simulink model "bai3c_pid"  (R2018a)
settings: Solver=VariableStepAuto  StartTime=0.0  StopTime=500  RelTol=1e-3
libraries: simulink x3
settings Model: Creator=MY PC  LastModifiedBy=Administrator
settings DataIOCC: ReturnWorkspaceOutputs=on
settings SFSimCC: SimUseLocalCustomCode=on
settings RTWCC: RTWUseLocalCustomCode=on

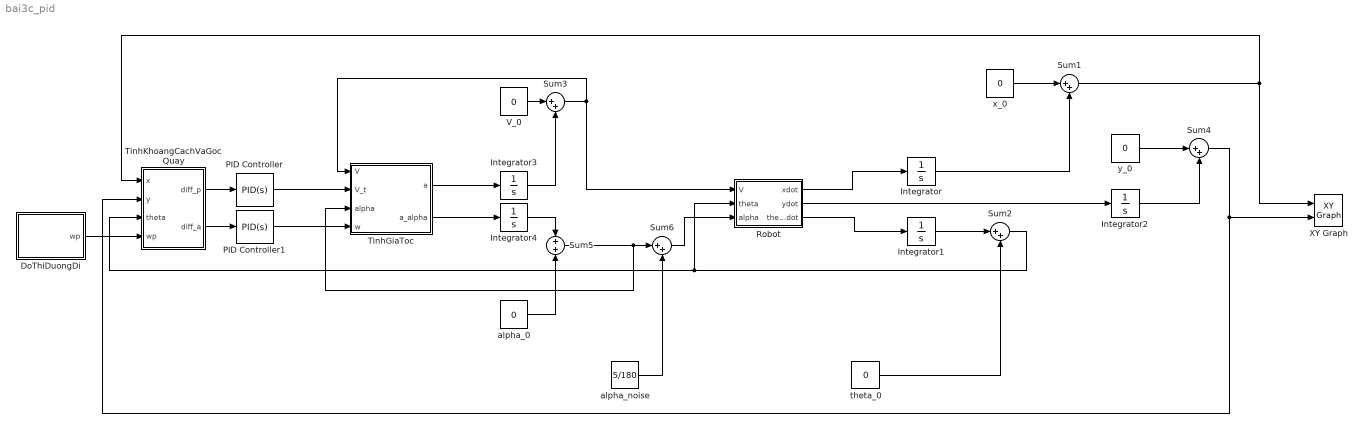
== system bai3c_pid ==
  DoThiDuongDi : MATLAB Function  TreatAsAtomicUnit=on
  Integrator{,1..4} (5 alike) : Integrator
  PID Controller : simulink/Continuous/PID Controller  Controller=PID  TimeDomain=Continuous-time  SampleTime=-1  IntegratorMethod=Forward Euler  FilterMethod=Forward Euler  Form=Parallel  UseFilter=on  ControllerParametersSource=internal  P=1/200  I=1/90000  D=0  N=1000000  InitialConditionSource=internal  InitialConditionForIntegrator=0  InitialConditionForFilter=0  ExternalReset=none  LimitOutput=off  UpperSaturationLimit=inf  LowerSaturationLimit=-inf  LinearizeAsGain=on  AntiWindupMode=none  Kb=1  TrackingMode=off  Kt=1  PParamMin=[]  PParamMax=[]  IParamMin=[]  IParamMax=[]  DParamMin=[]  DParamMax=[]  NParamMin=[]  NParamMax=[]  KbParamMin=[]  KbParamMax=[]  KtParamMin=[]  KtParamMax=[]  POutMin=[]  POutMax=[]  IOutMin=[]  IOutMax=[]  DOutMin=[]  DOutMax=[]  NOutMin=[]  NOutMax=[]  KbOutMin=[]  KbOutMax=[]  KtOutMin=[]  KtOutMax=[]  IntegratorOutMin=[]  IntegratorOutMax=[]  FilterOutMin=[]  FilterOutMax=[]  SumOutMin=[]  SumOutMax=[]  SumI1OutMin=[]  SumI1OutMax=[]  SumI2OutMin=[]  SumI2OutMax=[]  SumI3OutMin=[]  SumI3OutMax=[]  SumDOutMin=[]  SumDOutMax=[]  SaturationOutMin=[]  SaturationOutMax=[]  IntegratorContinuousStateAttributes=''  IntegratorStateMustResolveToSignalObject=off  IntegratorRTWStateStorageClass=Auto  FilterContinuousStateAttributes=''  FilterStateMustResolveToSignalObject=off  FilterRTWStateStorageClass=Auto  DifferentiatorICPrevScaledInput=0  DifferentiatorOutMin=[]  DifferentiatorOutMax=[]  FilterDiffOutCoefMin=[]  FilterDiffOutCoefMax=[]  SumDenOutMin=[]  SumDenOutMax=[]  SumNumOutMin=[]  SumNumOutMax=[]  ReciprocalOutMin=[]  ReciprocalOutMax=[]  DivideOutMin=[]  DivideOutMax=[]  TunerSelectOption=Transfer Function Based (PID Tuner App)
  PID Controller1 : simulink/Continuous/PID Controller  Controller=PID  TimeDomain=Continuous-time  SampleTime=-1  IntegratorMethod=Forward Euler  FilterMethod=Forward Euler  Form=Parallel  UseFilter=on  ControllerParametersSource=internal  P=1/10  I=0  D=0  N=10000  InitialConditionSource=internal  InitialConditionForIntegrator=0  InitialConditionForFilter=0  ExternalReset=none  LimitOutput=off  UpperSaturationLimit=inf  LowerSaturationLimit=-inf  LinearizeAsGain=on  AntiWindupMode=none  Kb=1  TrackingMode=off  Kt=1  PParamMin=[]  PParamMax=[]  IParamMin=[]  IParamMax=[]  DParamMin=[]  DParamMax=[]  NParamMin=[]  NParamMax=[]  KbParamMin=[]  KbParamMax=[]  KtParamMin=[]  KtParamMax=[]  POutMin=[]  POutMax=[]  IOutMin=[]  IOutMax=[]  DOutMin=[]  DOutMax=[]  NOutMin=[]  NOutMax=[]  KbOutMin=[]  KbOutMax=[]  KtOutMin=[]  KtOutMax=[]  IntegratorOutMin=[]  IntegratorOutMax=[]  FilterOutMin=[]  FilterOutMax=[]  SumOutMin=[]  SumOutMax=[]  SumI1OutMin=[]  SumI1OutMax=[]  SumI2OutMin=[]  SumI2OutMax=[]  SumI3OutMin=[]  SumI3OutMax=[]  SumDOutMin=[]  SumDOutMax=[]  SaturationOutMin=[]  SaturationOutMax=[]  IntegratorContinuousStateAttributes=''  IntegratorStateMustResolveToSignalObject=off  IntegratorRTWStateStorageClass=Auto  FilterContinuousStateAttributes=''  FilterStateMustResolveToSignalObject=off  FilterRTWStateStorageClass=Auto  DifferentiatorICPrevScaledInput=0  DifferentiatorOutMin=[]  DifferentiatorOutMax=[]  FilterDiffOutCoefMin=[]  FilterDiffOutCoefMax=[]  SumDenOutMin=[]  SumDenOutMax=[]  SumNumOutMin=[]  SumNumOutMax=[]  ReciprocalOutMin=[]  ReciprocalOutMax=[]  DivideOutMin=[]  DivideOutMax=[]  TunerSelectOption=Transfer Function Based (PID Tuner App)
  Robot : MATLAB Function  TreatAsAtomicUnit=on
  Sum{1..4,6} (5 alike) : Sum  Inputs=|++
  Sum5 : Sum
  TinhGiaToc : MATLAB Function  TreatAsAtomicUnit=on
  TinhKhoangCachVaGocQuay : MATLAB Function  TreatAsAtomicUnit=on
  V_0 : Constant  Value=0
  XY Graph : simulink/Sinks/XY Graph  xmin=-10  xmax=60  ymin=-10  ymax=5  st=-1
  alpha_0 : Constant  Value=0
  alpha_noise : Constant  Value=5/180
  theta_0 : Constant  Value=0
  x_0 : Constant  Value=0
  y_0 : Constant  Value=0
  wires:
  x_0/1 -> Sum1/1
  Integrator/1 -> Sum1/2
  Robot/1(xdot) -> Integrator/1
  Robot/2(ydot) -> Integrator2/1
  y_0/1 -> Sum4/1
  Integrator2/1 -> Sum4/2
  DoThiDuongDi/1(wp) -> TinhKhoangCachVaGocQuay/4(wp)
  TinhKhoangCachVaGocQuay/1(diff_p) -> PID Controller/1
  Sum1/1 -> XY Graph/1, TinhKhoangCachVaGocQuay/1(x)
  Sum4/1 -> XY Graph/2, TinhKhoangCachVaGocQuay/2(y)
  Integrator1/1 -> Sum2/1
  theta_0/1 -> Sum2/2
  Sum2/1 -> TinhKhoangCachVaGocQuay/3(theta), Robot/2(theta)
  TinhKhoangCachVaGocQuay/2(diff_a) -> PID Controller1/1
  Robot/3(thetadot) -> Integrator1/1
  V_0/1 -> Sum3/1
  Integrator3/1 -> Sum3/2
  TinhGiaToc/1(a) -> Integrator3/1
  Sum3/1 -> Robot/1(V), TinhGiaToc/1(V)
  TinhGiaToc/2(a_alpha) -> Integrator4/1
  alpha_0/1 -> Sum5/2
  Integrator4/1 -> Sum5/1
  Sum5/1 -> TinhGiaToc/3(alpha), Sum6/1
  alpha_noise/1 -> Sum6/2
  Sum6/1 -> Robot/3(alpha)
  PID Controller1/1 -> TinhGiaToc/4(w)
  PID Controller/1 -> TinhGiaToc/2(V_t)

== matlab function bai3c_pid/TinhKhoangCachVaGocQuay ==
  data: x input; diff_p output; y input; theta input; wp input; diff_a output
function [diff_p, diff_a]= fcn(x,y,theta,wp)
coder.extrinsic('wrapToPi');

% chọn điểm mục tiêu
if y>-4
    x_t = wp(16,1);
    y_t = wp(16,2);
    for i=1:15
        if wp(i,1)>x
            x_t = wp(i+2,1);
            y_t = wp(i+2,2);
            break
        end
    end
else
    x_t = 0;
    y_t = -8;
    for i=16:28
        if wp(i,1)<x
            x_t = wp(i+1,1);
            y_t = wp(i+1,2);
            break
        end
    end
end

% chuẩn hóa theta
while theta>2*pi
    theta = theta-2*pi;
end
while theta<-2*pi
    theta = theta+2*pi;
end
if theta<-pi
    theta = theta+2*pi;
elseif theta>pi
    theta = theta-2*pi;
end

% khoảng cách & góc lệch so với điểm mục tiêu
diff_p = (x_t-x)*(x_t-x) + (y_t-y)*(y_t-y);
a = atan2(y_t-y, x_t-x);

diff_a = a-theta;
if diff_a>pi
    diff_a = diff_a-2*pi;
elseif diff_a<-pi
    diff_a = diff_a+2*pi;
end

% a = atan2(y_t-y, x_t-x);
% t = theta;
%

== matlab function bai3c_pid/Robot ==
  data: V input; xdot output; theta input; ydot output; alpha input; thetadot output
function [xdot, ydot,thetadot]= fcn(V, theta, alpha)
if alpha>pi/4
    alpha = pi/4;
elseif alpha<-pi/4
    alpha = -pi/4;
end
if V>1.5+0.03*20
    V = 1.5+0.03*20;
elseif V<0
    V = 0;
end
coder.extrinsic('wrapToPi');
d = sqrt(4.5);
theta =  wrapToPi(theta);
xdot = zeros(1,1);
ydot = zeros(1,1);
xdot = V*cos(theta);
ydot = V*sin(theta);
if alpha==0
    thetadot = 0;
else
    R = d/tan(alpha);
    thetadot = zeros(1,1);
    thetadot = V/R;
end

== matlab function bai3c_pid/DoThiDuongDi ==
  data: wp output
function wp = fcn()
% tạo waypoints
X = linspace(0,20,10);
Y = zeros(1,10);
Z = [X;Y].';

X = linspace(20,0,10);
Y = -ones(1,10)*8;
Z2 = [X;Y].';

t = linspace(0, pi, 10);
X = 20 + 4*cos(pi/2-t);
Y = 4*cos(-t)-4;
Z3 = [X;Y].';

wp = [Z;Z3;Z2];

== matlab function bai3c_pid/TinhGiaToc ==
  data: V input; a output; V_t input; a_alpha output; alpha input; w input
function [a, a_alpha]= fcn(V, V_t, alpha, w)

% hàm chuẩn hóa
V = min(V,0.5);

Valpha = min(abs(Valpha),0.5)*sign(Valpha);

% Chuẩn hóa 
V = min(V,0.5);

Valpha = min(abs(Valpha),0.5)*sign(Valpha);

% dựa trên độ lệch so với điểm mục tiêu, tính gia tốc, tốc độ xoay alpha
if V_t>V
    a = min(V_t-V,0.3);
else
    a = -min(V-V_t,0.3);
end
d = sqrt(4.5);

alpha_t = pi/2 - atan2(V,d*w);
alpha = min(abs(alpha),pi/4)*sign(alpha);
if alpha_t>alpha
    a_alpha = min(alpha_t-alpha,0.3);
else
    a_alpha = -min(alpha-alpha_t,0.3);
end
